simulink model "TTypeInverter_R2022a"  (R2022a)
settings: Solver=ode23t  StartTime=0.0  StopTime=0.2  RelTol=1e-3  EnableMultiTasking=on
values from neighbouring files (symbols this model uses):
  C_c = 30*10^-6    (= 3e-05)    [TTypeInverterVals.m]
  den = abs(G_pr_r_z.Denominator{1,1})    [TTypeInverterVals.m]
  den15 = abs(G_pr_r_15_z.Denominator{1,1})    [TTypeInverterVals.m]
  den21 = abs(G_pr_r_21_z.Denominator{1,1})    [TTypeInverterVals.m]
  den5 = abs(G_pr_r_5_z.Denominator{1,1})    [TTypeInverterVals.m]
  den7 = abs(G_pr_r_7_z.Denominator{1,1})    [TTypeInverterVals.m]
  f_o = 50    [TTypeInverterVals.m]
  G_diff_z = c2d(G_diff_s,Ts,opt)    [ControllerDesign.m]    (also in TTypeInverterVals.m = c2d(G_diff_s,Ts,'foh'))
  Kc = 2.5    [ControllerDesign.m]    (also in TTypeInverterVals.m)
  Klim = 5    [TTypeInverterVals.m]
  Kp = 1/mag/(10^(1.14/20))    [ControllerDesign.m]    (also in TTypeInverterVals.m = 0.9444)
  Kr = omega_c_o/2    (= 3141.59265359)    [ControllerDesign.m]    (also in TTypeInverterVals.m)
  N = 26    [Inductance.m]    (also in TTypeInverterVals.m = [0])
  num = abs(G_pr_r_z.Numerator{1,1})    [TTypeInverterVals.m]
  num15 = abs(G_pr_r_15_z.Numerator{1,1})    [TTypeInverterVals.m]
  num21 = abs(G_pr_r_21_z.Numerator{1,1})    [TTypeInverterVals.m]
  num5 = abs(G_pr_r_5_z.Numerator{1,1})    [TTypeInverterVals.m]
  num7 = abs(G_pr_r_7_z.Numerator{1,1})    [TTypeInverterVals.m]
  omega_o = fo*2*pi    (= 314.159265359)    [ControllerDesign.m]    (also in TTypeInverterVals.m)
  omega_w = 0.1*2*pi    (= 0.628318530718)    [ControllerDesign.m]    (also in TTypeInverterVals.m)
  pr_sat_val = ceil(3*io_nom)    [TTypeInverterVals.m]
  Q = eye(3)    [TTypeInverterVals.m]
  R = [R_iL 0 ... (first row only)    [TTypeInverterVals.m]
  R_l_20p = Vout^2/P_lin_20p    (= 10.58)    [TTypeInverterVals.m]
  R_l_3p = Vout/(P_max_3p/(Vout*3))    (= 2.116)    [TTypeInverterVals.m]
  R_l_80p = Vout^2/P_lin_80p    (= 2.645)    [TTypeInverterVals.m]
  R_l_nl = Vout^2/P_lin    (= 3.11176470588)    [TTypeInverterVals.m]
  R_l_nl_3p = Vout_3p^2/P_lin_3p    [TTypeInverterVals.m]
  R_Lc = 5.6e-3    (= 0.0056)    [TTypeInverterVals.m]
  R_nl_load = Uc^2/(0.66*S_tot)    (= 14.9121893939)    [TTypeInverterVals.m]
  R_nl_load_3p = Uc_3p^2/(0.66*S_tot_3p)    (= 4.97072979798)    [TTypeInverterVals.m]
  R_nl_s = 0.04*Vout^2/S_tot    (= 0.2645)    [TTypeInverterVals.m]
  R_nl_s_3p = 0.04*Vout_3p^2/S_tot_3p    [TTypeInverterVals.m]
  T_sw = 1/f_sw    (= 4.16666666667e-05)    [TTypeInverterVals.m]
  Tcomp = Ts/4    (= 2.60400009204e-06)    [TTypeInverterVals.m]
  Ts = 1/fs    (= 1.04166666667e-05)    [ControllerDesign.m]    (also in KalmanFilter.m = 2.08333333333e-05; TTypeInverterVals.m = 1.04160003681e-05)
  VDC = 800    [TTypeInverterVals.m]
  Vout_amp = Vout*sqrt(2)    [TTypeInverterVals.m]
undefined symbols (not defined in the file or in its folder): a0, a1, b0, b1, Discrete, G_ll_z, Ki, Kpc, KT, kv, Time, UKF_data
libraries: ee_lib x94, nesl_utility x48, fl_lib x39, dspstat3 x15, spsTriangleGeneratorLib x6, ctrlSharedLib x3, spsRMSLib x3, spsTHDLib x3
(part 5 of 5)

== system TTypeInverter_R2022a/Phase 3/Controllers/Voltage Controller/Third Harmonic ==
  In : Inport
  Anti-Windup : Inport  Port=2
  1/b0 : Gain  Gain=1/(KT(2)*KT(2)+2*omega_w(2)*KT(2)+3*3*omega_o*omega_o)
  Delay1 : Delay  DelayLength=1  SampleTime=Ts
  Delay3 : Delay  SampleTime=Ts
  Delay4 : Delay  DelayLength=1  SampleTime=Ts
  Delay5 : Delay  DelayLength=1  SampleTime=Ts
  Klim : Gain  Gain=Klim
  Sum : Sum  Inputs=|+-
  Sum3 : Sum  Inputs=|+-
  Sum4 : Sum  Inputs=|++
  Sum5 : Sum  Inputs=+-|
  a1 : Gain  Gain=2*Kr(2)*KT(2)*omega_w(2)
  b1 : Gain  Gain=2*KT(2)*KT(2)-2*3*3*omega_o*omega_o
  b2 : Gain  Gain=KT(2)*KT(2)+2*omega_w(2)*KT(2)-3*3*omega_o*omega_o
  Out : Outport
  wires:
  Delay3/1 -> Sum3/2  "e(n-2)"
  Delay5/1 -> b2/1  "y(n-2)"
  Klim/1 -> Sum/2
  1/b0/1 -> Out/1, Delay4/1  "y(n)"
  a1/1 -> Sum4/1
  Sum4/1 -> 1/b0/1
  Sum3/1 -> a1/1
  b2/1 -> Sum5/2
  Sum5/1 -> Sum4/2
  Sum/1 -> Sum3/1, Delay3/1  "e(n)"
  b1/1 -> Sum5/1
  Delay4/1 -> Delay5/1, b1/1  "y(n-1)"
  In/1 -> Sum/1
  Delay1/1 -> Klim/1
  Anti-Windup/1 -> Delay1/1

== matlab function TTypeInverter_R2022a/Phase 3/Kalman Filter - Unscented/Unscented Kalman Filter/Update Step ==
  data: y input; yhat_minus input; P_minus input; xhat_minus input; yhat output; xhat output; UKF_struct parameter; P output
function [yhat, xhat, P] = fcn(y, yhat_minus, P_minus, xhat_minus, UKF_struct)


% 1) Calculate Kalman gain
Lk = ( P_minus*(UKF_struct.C') ) * inv( UKF_struct.C*P_minus*(UKF_struct.C') + UKF_struct.R );


% 2) Update predictions
xhat = xhat_minus + Lk*(y-yhat_minus);
yhat = UKF_struct.C * xhat;


% 3) Update error covariance
P = (eye(length(P_minus)) - Lk*UKF_struct.C)*P_minus;

== matlab function TTypeInverter_R2022a/Phase 1/Kalman Filter - Unscented/Unscented Kalman Filter/Predict Step ==
  data: yhat_minus output; xhat_k input; P_k input; P_minus output; u_k input; xhat_minus output; UKF_struct parameter
function [yhat_minus, P_minus, xhat_minus] = fcn(xhat_k, P_k, u_k, UKF_struct)

% For testing with and without including the mean value
calc = 'WithoutMean';

if strcmp(calc,'WithoutMean')
    n = 2*UKF_struct.n;
    w = 1/(2*(UKF_struct.n+UKF_struct.kappa))*ones(n,1);
elseif strcmp(calc, 'WithMean')
    n = 2*UKF_struct.n+1;
    w = [0.5*ones(length(xhat_k),1); UKF_struct.kappa; 0.5*ones(length(xhat_k),1)]/(UKF_struct.n+UKF_struct.kappa);
else
    disp('Calculation type error in Unscented Kalman filter')
end


% Initialize variables
x_sigma = zeros(length(xhat_k), n);
xhat_sigma = zeros(length(xhat_k), n);
yhat_minus = zeros(height(UKF_struct.C), 1);


% 1) Calculate x-sigma points (xhat sigmas)
P_k_sqrt = real(sqrtm((UKF_struct.n+UKF_struct.kappa)*P_k));
for i = 1:length(xhat_k)
    x_sigma(:,i) = xhat_k(:) + P_k_sqrt(:,i);
    if strcmp(calc,'WithoutMean')
        x_sigma(:,i+UKF_struct.n) = xhat_k(:) - P_k_sqrt(:,i);
    elseif strcmp(calc,'WithMean')
        x_sigma(:,i+UKF_struct.n+1) = xhat_k(:) - P_k_sqrt(:,i);
        x_sigma(:,UKF_struct.n+1) = xhat_k(:);
    end
end


% 2) Calculate y-sigma points (xhat_minus sigmas)
for i = 1:n
    xhat_sigma(:,i) = [x_sigma(1,i) + UKF_struct.Ts*( ((2.2737*abs(x_sigma(1,i)))^1.9167+44052.86)/3.9813 * (u_k(1) - x_sigma(1,i)*UKF_struct.RLc - x_sigma(3,i)*UKF_struct.RCc - x_sigma(2,i)) ); ...
                       x_sigma(2,i) + UKF_struct.Ts*x_sigma(3,i)/UKF_struct.Cc; ...
                       x_sigma(1,i) - u_k(2)];

                       % Calculate ic from next iL - io
                       % x_sigma(1,i) + UKF_struct.Ts*( ((2.2737*abs(x_sigma(1,i)))^1.9167+44052.86)/3.9813 * (u_k(1) - x_sigma(1,i)*UKF_struct.RLc - x_sigma(3,i)*UKF_struct.RCc - x_sigma(2,i)) ) - u_k(2)];
                       
                       % Calculate ic by taking diL and calculating dio
                       %x_sigma(3,i) + UKF_struct.Ts*UKF_struct.Cc*(x_sigma(1,i)+(1/UKF_struct.Lg)*(x_sigma(2,i) - u_k(2)*UKF_struct.RLg + x_sigma(3,i)*UKF_struct.RCc) )];
                       
                       % Calculate ic by calculating both diL and dio
                       %x_sigma(3,i) + UKF_struct.Ts*UKF_struct.Cc*( ((2.2737*abs(x_sigma(1,i)))^1.9167+44052.86)/3.9813 * (u_k(1) - x_sigma(1,i)*UKF_struct.RLc - x_sigma(3,i)*UKF_struct.RCc - x_sigma(2,i)) ...
                       %- (1/UKF_struct.Lg)*(x_sigma(2,i) - u_k(2)*UKF_struct.RLg + x_sigma(3,i)*UKF_struct.RCc) )];
end


% 3) Predict states and outputs
xhat_minus = xhat_sigma*w;

yhat_minus(1) = xhat_minus(1);
yhat_minus(2) = xhat_minus(2) + xhat_minus(3)*UKF_struct.RCc;


% 4) Predict error covariance
P_minus = (xhat_sigma-xhat_minus)*diag(w)*(xhat_sigma-xhat_minus)' + UKF_struct.Q;


% Standard Kalman filter implementation
%xhat_minus = xhat_k + UKF_struct.Ts * (UKF_struct.A*xhat_k + UKF_struct.B*u_k);
%yhat_minus = UKF_struct.C*xhat_minus;
%P_minus = UKF_struct.A*P_k*(UKF_struct.A') + UKF_struct.Q;

== matlab function TTypeInverter_R2022a/Phase 1/Controllers/Current Controller/Variable Gain ==
  data: iL input; e_out output; e_in input
function e_out = fcn(iL, e_in)

% Create gain that somewhat follows the inductance graph (by linearization)
if abs(iL)<=218
    e_out = e_in - e_in*abs(iL)*1/218;
else
    e_out = 0;
end

== matlab function TTypeInverter_R2022a/Phase 1/Kalman Filter - Unscented/Unscented Kalman Filter/Update Step ==
  data: y input; yhat_minus input; P_minus input; xhat_minus input; yhat output; xhat output; UKF_struct parameter; P output
function [yhat, xhat, P] = fcn(y, yhat_minus, P_minus, xhat_minus, UKF_struct)


% 1) Calculate Kalman gain
Lk = ( P_minus*(UKF_struct.C') ) * inv( UKF_struct.C*P_minus*(UKF_struct.C') + UKF_struct.R );


% 2) Update predictions
xhat = xhat_minus + Lk*(y-yhat_minus);
yhat = UKF_struct.C * xhat;


% 3) Update error covariance
P = (eye(length(P_minus)) - Lk*UKF_struct.C)*P_minus;

== matlab function TTypeInverter_R2022a/Phase 2/Controllers/Current Controller/Variable Gain ==
  data: iL input; e_out output; e_in input
function e_out = fcn(iL, e_in)

% Create gain that somewhat follows the inductance graph (by linearization)
if abs(iL)<=218
    e_out = e_in - e_in*abs(iL)*1/218;
else
    e_out = 0;
end

== matlab function TTypeInverter_R2022a/Phase 2/Kalman Filter - Unscented/Unscented Kalman Filter/Predict Step ==
  data: yhat_minus output; xhat_k input; P_k input; P_minus output; u_k input; xhat_minus output; UKF_struct parameter
function [yhat_minus, P_minus, xhat_minus] = fcn(xhat_k, P_k, u_k, UKF_struct)

% For testing with and without including the mean value
calc = 'WithoutMean';

if strcmp(calc,'WithoutMean')
    n = 2*UKF_struct.n;
    w = 1/(2*(UKF_struct.n+UKF_struct.kappa))*ones(n,1);
elseif strcmp(calc, 'WithMean')
    n = 2*UKF_struct.n+1;
    w = [0.5*ones(length(xhat_k),1); UKF_struct.kappa; 0.5*ones(length(xhat_k),1)]/(UKF_struct.n+UKF_struct.kappa);
else
    disp('Calculation type error in Unscented Kalman filter')
end


% Initialize variables
x_sigma = zeros(length(xhat_k), n);
xhat_sigma = zeros(length(xhat_k), n);
yhat_minus = zeros(height(UKF_struct.C), 1);


% 1) Calculate x-sigma points (xhat sigmas)
P_k_sqrt = real(sqrtm((UKF_struct.n+UKF_struct.kappa)*P_k));
for i = 1:length(xhat_k)
    x_sigma(:,i) = xhat_k(:) + P_k_sqrt(:,i);
    if strcmp(calc,'WithoutMean')
        x_sigma(:,i+UKF_struct.n) = xhat_k(:) - P_k_sqrt(:,i);
    elseif strcmp(calc,'WithMean')
        x_sigma(:,i+UKF_struct.n+1) = xhat_k(:) - P_k_sqrt(:,i);
        x_sigma(:,UKF_struct.n+1) = xhat_k(:);
    end
end


% 2) Calculate y-sigma points (xhat_minus sigmas)
for i = 1:n
    xhat_sigma(:,i) = [x_sigma(1,i) + UKF_struct.Ts*( ((2.2737*abs(x_sigma(1,i)))^1.9167+44052.86)/3.9813 * (u_k(1) - x_sigma(1,i)*UKF_struct.RLc - x_sigma(3,i)*UKF_struct.RCc - x_sigma(2,i)) ); ...
                       x_sigma(2,i) + UKF_struct.Ts*x_sigma(3,i)/UKF_struct.Cc; ...
                       x_sigma(1,i) - u_k(2)];

                       % Calculate ic from next iL - io
                       % x_sigma(1,i) + UKF_struct.Ts*( ((2.2737*abs(x_sigma(1,i)))^1.9167+44052.86)/3.9813 * (u_k(1) - x_sigma(1,i)*UKF_struct.RLc - x_sigma(3,i)*UKF_struct.RCc - x_sigma(2,i)) ) - u_k(2)];
                       
                       % Calculate ic by taking diL and calculating dio
                       %x_sigma(3,i) + UKF_struct.Ts*UKF_struct.Cc*(x_sigma(1,i)+(1/UKF_struct.Lg)*(x_sigma(2,i) - u_k(2)*UKF_struct.RLg + x_sigma(3,i)*UKF_struct.RCc) )];
                       
                       % Calculate ic by calculating both diL and dio
                       %x_sigma(3,i) + UKF_struct.Ts*UKF_struct.Cc*( ((2.2737*abs(x_sigma(1,i)))^1.9167+44052.86)/3.9813 * (u_k(1) - x_sigma(1,i)*UKF_struct.RLc - x_sigma(3,i)*UKF_struct.RCc - x_sigma(2,i)) ...
                       %- (1/UKF_struct.Lg)*(x_sigma(2,i) - u_k(2)*UKF_struct.RLg + x_sigma(3,i)*UKF_struct.RCc) )];
end


% 3) Predict states and outputs
xhat_minus = xhat_sigma*w;

yhat_minus(1) = xhat_minus(1);
yhat_minus(2) = xhat_minus(2) + xhat_minus(3)*UKF_struct.RCc;


% 4) Predict error covariance
P_minus = (xhat_sigma-xhat_minus)*diag(w)*(xhat_sigma-xhat_minus)' + UKF_struct.Q;


% Standard Kalman filter implementation
%xhat_minus = xhat_k + UKF_struct.Ts * (UKF_struct.A*xhat_k + UKF_struct.B*u_k);
%yhat_minus = UKF_struct.C*xhat_minus;
%P_minus = UKF_struct.A*P_k*(UKF_struct.A') + UKF_struct.Q;

== matlab function TTypeInverter_R2022a/Phase 2/Kalman Filter - Unscented/Unscented Kalman Filter/Update Step ==
  data: y input; yhat_minus input; P_minus input; xhat_minus input; yhat output; xhat output; UKF_struct parameter; P output
function [yhat, xhat, P] = fcn(y, yhat_minus, P_minus, xhat_minus, UKF_struct)


% 1) Calculate Kalman gain
Lk = ( P_minus*(UKF_struct.C') ) * inv( UKF_struct.C*P_minus*(UKF_struct.C') + UKF_struct.R );


% 2) Update predictions
xhat = xhat_minus + Lk*(y-yhat_minus);
yhat = UKF_struct.C * xhat;


% 3) Update error covariance
P = (eye(length(P_minus)) - Lk*UKF_struct.C)*P_minus;

== matlab function TTypeInverter_R2022a/Phase 3/Controllers/Current Controller/Variable Gain ==
  data: iL input; e_out output; e_in input
function e_out = fcn(iL, e_in)

% Create gain that somewhat follows the inductance graph (by linearization)
if abs(iL)<=218
    e_out = e_in - e_in*abs(iL)*1/218;
else
    e_out = 0;
end

== matlab function TTypeInverter_R2022a/Phase 3/Kalman Filter - Unscented/Unscented Kalman Filter/Predict Step ==
  data: yhat_minus output; xhat_k input; P_k input; P_minus output; u_k input; xhat_minus output; UKF_struct parameter
function [yhat_minus, P_minus, xhat_minus] = fcn(xhat_k, P_k, u_k, UKF_struct)

% For testing with and without including the mean value
calc = 'WithoutMean';

if strcmp(calc,'WithoutMean')
    n = 2*UKF_struct.n;
    w = 1/(2*(UKF_struct.n+UKF_struct.kappa))*ones(n,1);
elseif strcmp(calc, 'WithMean')
    n = 2*UKF_struct.n+1;
    w = [0.5*ones(length(xhat_k),1); UKF_struct.kappa; 0.5*ones(length(xhat_k),1)]/(UKF_struct.n+UKF_struct.kappa);
else
    disp('Calculation type error in Unscented Kalman filter')
end


% Initialize variables
x_sigma = zeros(length(xhat_k), n);
xhat_sigma = zeros(length(xhat_k), n);
yhat_minus = zeros(height(UKF_struct.C), 1);


% 1) Calculate x-sigma points (xhat sigmas)
P_k_sqrt = real(sqrtm((UKF_struct.n+UKF_struct.kappa)*P_k));
for i = 1:length(xhat_k)
    x_sigma(:,i) = xhat_k(:) + P_k_sqrt(:,i);
    if strcmp(calc,'WithoutMean')
        x_sigma(:,i+UKF_struct.n) = xhat_k(:) - P_k_sqrt(:,i);
    elseif strcmp(calc,'WithMean')
        x_sigma(:,i+UKF_struct.n+1) = xhat_k(:) - P_k_sqrt(:,i);
        x_sigma(:,UKF_struct.n+1) = xhat_k(:);
    end
end


% 2) Calculate y-sigma points (xhat_minus sigmas)
for i = 1:n
    xhat_sigma(:,i) = [x_sigma(1,i) + UKF_struct.Ts*( ((2.2737*abs(x_sigma(1,i)))^1.9167+44052.86)/3.9813 * (u_k(1) - x_sigma(1,i)*UKF_struct.RLc - x_sigma(3,i)*UKF_struct.RCc - x_sigma(2,i)) ); ...
                       x_sigma(2,i) + UKF_struct.Ts*x_sigma(3,i)/UKF_struct.Cc; ...
                       x_sigma(1,i) - u_k(2)];

                       % Calculate ic from next iL - io
                       % x_sigma(1,i) + UKF_struct.Ts*( ((2.2737*abs(x_sigma(1,i)))^1.9167+44052.86)/3.9813 * (u_k(1) - x_sigma(1,i)*UKF_struct.RLc - x_sigma(3,i)*UKF_struct.RCc - x_sigma(2,i)) ) - u_k(2)];
                       
                       % Calculate ic by taking diL and calculating dio
                       %x_sigma(3,i) + UKF_struct.Ts*UKF_struct.Cc*(x_sigma(1,i)+(1/UKF_struct.Lg)*(x_sigma(2,i) - u_k(2)*UKF_struct.RLg + x_sigma(3,i)*UKF_struct.RCc) )];
                       
                       % Calculate ic by calculating both diL and dio
                       %x_sigma(3,i) + UKF_struct.Ts*UKF_struct.Cc*( ((2.2737*abs(x_sigma(1,i)))^1.9167+44052.86)/3.9813 * (u_k(1) - x_sigma(1,i)*UKF_struct.RLc - x_sigma(3,i)*UKF_struct.RCc - x_sigma(2,i)) ...
                       %- (1/UKF_struct.Lg)*(x_sigma(2,i) - u_k(2)*UKF_struct.RLg + x_sigma(3,i)*UKF_struct.RCc) )];
end


% 3) Predict states and outputs
xhat_minus = xhat_sigma*w;

yhat_minus(1) = xhat_minus(1);
yhat_minus(2) = xhat_minus(2) + xhat_minus(3)*UKF_struct.RCc;


% 4) Predict error covariance
P_minus = (xhat_sigma-xhat_minus)*diag(w)*(xhat_sigma-xhat_minus)' + UKF_struct.Q;


% Standard Kalman filter implementation
%xhat_minus = xhat_k + UKF_struct.Ts * (UKF_struct.A*xhat_k + UKF_struct.B*u_k);
%yhat_minus = UKF_struct.C*xhat_minus;
%P_minus = UKF_struct.A*P_k*(UKF_struct.A') + UKF_struct.Q;
